simulink library "exampleMicrogridLibrary"  (R2017b)
settings: Solver=VariableStepAuto  StartTime=0.0  StopTime=10.0  RelTol=1e-3
undefined symbols (not defined in the file): BR, D1, Delta, DiscIntNeverNeededParam, Fnom, gcbh, Ion, kv, Lithium, Ls, Rs, sps_rtmsupport, StationData, Ts, Ts_Control, Vrms
libraries: powerlib x75, simulink x29, powerlib_meascontrol x26, sps_avr x5, spsDieselMotorModel x3, electricdrivelib x2, re_lib x1
(part 5 of 5)

== system exampleMicrogridLibrary/Solar Array (EMT Model)/Inverter Control/Current Regulator ==
  note: Current Regulator
      | ================
  note: Sign Convention: Current going out of the converter = positive current
  note: Iq positive --> The converter absorbs reactive power ("Inductive mode") = Reactive Power Q negative
  note: Id positive --> The converter generates active power ("Inverter mode") = Active Power P positive
  VdVq_meas : Inport  PortDimensions=2
  IdIq_meas : Inport  Port=2  PortDimensions=2
  IdIq_ref : Inport  Port=3  PortDimensions=2
  Add1 : Sum  Inputs=++-
  Add2 : Sum
  Add3 : Sum  Inputs=+++
  Demux : Demux  Outputs=2
  Demux1 : Demux  Outputs=2
  Lff : Gain  Gain=Ltot_pu  SaturateOnIntegerOverflow=on  OutDataTypeStr=Inherit: Same as input  ParamDataTypeStr=Inherit: Same as input
  "Lff  " : Gain  Gain=Ltot_pu  SaturateOnIntegerOverflow=on  OutDataTypeStr=Inherit: Same as input  ParamDataTypeStr=Inherit: Same as input
  Mux : Mux  Inputs=2
  PI : simulink/Continuous/PID Controller  Controller=PI  TimeDomain=Discrete-time  SampleTime=Ts_Control  IntegratorMethod=Forward Euler  FilterMethod=Forward Euler  Form=Parallel  UseFilter=on  ControllerParametersSource=internal  P=Kp_Ireg  I=Ki_Ireg  D=0  N=100  InitialConditionSource=internal  InitialConditionForIntegrator=0  InitialConditionForFilter=0  ExternalReset=none  LimitOutput=on  UpperSaturationLimit=1.5  LowerSaturationLimit=-1.5  LinearizeAsGain=off  AntiWindupMode=none  Kb=1  TrackingMode=off  Kt=1  PParamMin=[]  PParamMax=[]  IParamMin=[]  IParamMax=[]  DParamMin=[]  DParamMax=[]  NParamMin=[]  NParamMax=[]  KbParamMin=[]  KbParamMax=[]  KtParamMin=[]  KtParamMax=[]  POutMin=[]  POutMax=[]  IOutMin=[]  IOutMax=[]  DOutMin=[]  DOutMax=[]  NOutMin=[]  NOutMax=[]  KbOutMin=[]  KbOutMax=[]  KtOutMin=[]  KtOutMax=[]  IntegratorOutMin=[]  IntegratorOutMax=[]  FilterOutMin=[]  FilterOutMax=[]  SumOutMin=[]  SumOutMax=[]  SumI1OutMin=[]  SumI1OutMax=[]  SumI2OutMin=[]  SumI2OutMax=[]  SumI3OutMin=[]  SumI3OutMax=[]  SumDOutMin=[]  SumDOutMax=[]  SaturationOutMin=[]  SaturationOutMax=[]  IntegratorContinuousStateAttributes=''  IntegratorStateMustResolveToSignalObject=off  IntegratorRTWStateStorageClass=Auto  FilterContinuousStateAttributes=''  FilterStateMustResolveToSignalObject=off  FilterRTWStateStorageClass=Auto  DifferentiatorICPrevScaledInput=0  DifferentiatorOutMin=[]  DifferentiatorOutMax=[]  InitialConditionSetting=State (most efficient)  FilterDiffOutCoefMin=[]  FilterDiffOutCoefMax=[]  SumDenOutMin=[]  SumDenOutMax=[]  SumNumOutMin=[]  SumNumOutMax=[]  ReciprocalOutMin=[]  ReciprocalOutMax=[]  DivideOutMin=[]  DivideOutMax=[]  TunerSelectOption=Transfer Function Based (PID Tuner App)
  Rff : Gain  Gain=Rtot_pu  SaturateOnIntegerOverflow=on  OutDataTypeStr=Inherit: Same as input  ParamDataTypeStr=Inherit: Same as input
  "Rff " : Gain  Gain=Rtot_pu  SaturateOnIntegerOverflow=on  OutDataTypeStr=Inherit: Same as input  ParamDataTypeStr=Inherit: Same as input
  Saturation : Saturate  UpperLimit=1.5  LowerLimit=-1.5
  Sum : Sum  Inputs=|-+
  VdVq_conv : Outport
  wires:
  Mux/1 -> Add2/2
  PI/1 -> Add2/1  "PI"
  Sum/1 -> PI/1
  IdIq_ref/1 -> Sum/2, Demux1/1
  IdIq_meas/1 -> Sum/1
  Add2/1 -> Saturation/1
  Saturation/1 -> VdVq_conv/1
  VdVq_meas/1 -> Demux/1
  Demux/1 -> Add1/1
  "Rff "/1 -> Add1/2
  Demux1/1 -> "Rff "/1, Lff/1
  "Lff  "/1 -> Add1/3
  Demux1/2 -> "Lff  "/1, Rff/1
  Rff/1 -> Add3/2
  Lff/1 -> Add3/3
  Add1/1 -> Mux/1  "Feedforward"
  Demux/2 -> Add3/1
  Add3/1 -> Mux/2

== system exampleMicrogridLibrary/Solar Array (EMT Model)/Inverter Control/MPPT Parameters ==
  note: Parameters for Perturb and Observe Algorithm:
  note: Lower limit for Vdc_ref (Dmax)
  note: Initial value for Vdc_ref output (Dinit)
  note: Increment value used to increase/decrease Vdc_ref (DeltaD)
  note: Upper limit for Vdc_ref (Dmax)
  Iph_ : Constant  Value=Vnom_dc
  Iph_1 : Constant  Value=Limits_MPPT(1)
  Iph_2 : Constant  Value=Limits_MPPT(2)
  Iph_3 : Constant  Value=Increment_MPPT
  Mux : Mux
  Param : Outport
  wires:
  Mux/1 -> Param/1
  Iph_3/1 -> Mux/4
  Iph_2/1 -> Mux/3
  Iph_1/1 -> Mux/2
  Iph_/1 -> Mux/1

== system exampleMicrogridLibrary/Solar Array (EMT Model)/Inverter Control/PLL & Measurements ==
  note: PLL & Measurements
      | ===================
  Vabc_prim : Inport
  Iabc_prim : Inport  Port=2
  PLL (3ph) : powerlib_meascontrol/PLL/PLL (3ph)  Fmin=45  Par_Init="[-0.57  Fnom]"  ParK=[180, 3200, 1]  TcD=Ts  MaxRateChangeFreq=12  FilterCutOffFreq=25  Ts=Ts  AGC=on
  Selector1 : Selector  InputPortWidth=3  IndexOptions=Index vector (dialog)  Indices=[1 2]  OutputSizes=1
  Selector2 : Selector  InputPortWidth=3  IndexOptions=Index vector (dialog)  Indices=[1 2]  OutputSizes=1
  Terminator : Terminator
  V->pu : Gain  Gain=1/(Vnom_prim*sqrt(2)/sqrt(3))  SaturateOnIntegerOverflow=on  OutDataTypeStr=Inherit: Same as input  ParamDataTypeStr=Inherit: Same as input
  V->pu1 : Gain  Gain=Vnom_prim*sqrt(3)/Pnom/sqrt(2)  SaturateOnIntegerOverflow=on  OutDataTypeStr=Inherit: Same as input  ParamDataTypeStr=Inherit: Same as input
  abc to dq0 : powerlib_meascontrol/Transformations/abc to dq0  Alignment=90 degrees behind phase A axis
  abc to dq1 : powerlib_meascontrol/Transformations/abc to dq0  Alignment=90 degrees behind phase A axis
  wt : Outport
  VdVq_prim : Outport  Port=2
  IdIq_prim : Outport  Port=3
  wires:
  V->pu1/1 -> abc to dq1/1
  V->pu/1 -> PLL (3ph)/1, abc to dq0/1
  abc to dq1/1 -> Selector1/1
  Vabc_prim/1 -> V->pu/1
  Iabc_prim/1 -> V->pu1/1
  abc to dq0/1 -> Selector2/1
  Selector2/1 -> VdVq_prim/1
  Selector1/1 -> IdIq_prim/1
  PLL (3ph)/2 -> wt/1, abc to dq1/2, abc to dq0/2
  PLL (3ph)/1 -> Terminator/1

== system exampleMicrogridLibrary/Solar Array (EMT Model)/Inverter Control/Uabc_ref Generation max (m) = 1 ==
  note: (Correction for transformer
      |  D1 connection)
  note: (Correction for delai of Ts_Control)
  note: Uref Generation
      | ==============
  wt : Inport
  VdVq_conv : Inport  Port=2
  Add1 : Sum  Inputs=++++
  Add2 : Sum
  Complex to Magnitude-Angle : ComplexToMagnitudeAngle
  Constant : Constant  Value=-pi/6
  Constant1 : Constant  Value=Vnom_dc
  Constant2 : Constant  Value="[ 0  -2*pi/3  2*pi/3  ]"
  Constant3 : Constant  Value=Vnom_sec*sqrt(2)/sqrt(3)
  Constant4 : Constant  Value=Ts_Control*Fnom*(2*pi)
  Demux1 : Demux  Outputs=2
  Gain1 : Gain  Gain=1/2
  Product : Product  Inputs=*/  RndMeth=Zero
  Product1 : Product  Inputs=*/  RndMeth=Zero
  Product2 : Product  Inputs=**  RndMeth=Zero
  Real-Imag to Complex : RealImagToComplex
  Trigonometric Function : Trigonometry
  Uabc_ref : Outport
  wires:
  Constant1/1 -> Gain1/1
  VdVq_conv/1 -> Product1/1
  Product1/1 -> Demux1/1
  Gain1/1 -> Product/1
  Real-Imag to Complex/1 -> Complex to Magnitude-Angle/1
  Demux1/1 -> Real-Imag to Complex/1
  Demux1/2 -> Real-Imag to Complex/2
  Constant2/1 -> Add1/2
  Constant/1 -> Add1/3
  Constant3/1 -> Product/2
  Product/1 -> Product1/2
  Complex to Magnitude-Angle/2 -> Add2/1
  Add1/1 -> Add2/2
  Add2/1 -> Trigonometric Function/1
  Complex to Magnitude-Angle/1 -> Product2/1
  Trigonometric Function/1 -> Product2/2
  Product2/1 -> Uabc_ref/1
  wt/1 -> Add1/1
  Constant4/1 -> Add1/4

== system exampleMicrogridLibrary/Solar Array (EMT Model)/Inverter Control/VDC Regulator ==
  Vdc_meas : Inport  PortDimensions=1
  Vdc_ref : Inport  Port=2  PortDimensions=1
  PI : simulink/Continuous/PID Controller  Controller=PI  TimeDomain=Discrete-time  SampleTime=Ts_Control  IntegratorMethod=Trapezoidal  FilterMethod=Forward Euler  Form=Parallel  UseFilter=on  ControllerParametersSource=internal  P=Kp_VDCreg  I=Ki_VDCreg  D=0  N=100  InitialConditionSource=internal  InitialConditionForIntegrator=1  InitialConditionForFilter=0  ExternalReset=none  LimitOutput=on  UpperSaturationLimit=1.5  LowerSaturationLimit=-1.5  LinearizeAsGain=off  AntiWindupMode=none  Kb=1  TrackingMode=off  Kt=1  PParamMin=[]  PParamMax=[]  IParamMin=[]  IParamMax=[]  DParamMin=[]  DParamMax=[]  NParamMin=[]  NParamMax=[]  KbParamMin=[]  KbParamMax=[]  KtParamMin=[]  KtParamMax=[]  POutMin=[]  POutMax=[]  IOutMin=[]  IOutMax=[]  DOutMin=[]  DOutMax=[]  NOutMin=[]  NOutMax=[]  KbOutMin=[]  KbOutMax=[]  KtOutMin=[]  KtOutMax=[]  IntegratorOutMin=[]  IntegratorOutMax=[]  FilterOutMin=[]  FilterOutMax=[]  SumOutMin=[]  SumOutMax=[]  SumI1OutMin=[]  SumI1OutMax=[]  SumI2OutMin=[]  SumI2OutMax=[]  SumI3OutMin=[]  SumI3OutMax=[]  SumDOutMin=[]  SumDOutMax=[]  SaturationOutMin=[]  SaturationOutMax=[]  IntegratorContinuousStateAttributes=''  IntegratorStateMustResolveToSignalObject=off  IntegratorRTWStateStorageClass=Auto  FilterContinuousStateAttributes=''  FilterStateMustResolveToSignalObject=off  FilterRTWStateStorageClass=Auto  DifferentiatorICPrevScaledInput=0  DifferentiatorOutMin=[]  DifferentiatorOutMax=[]  InitialConditionSetting=State (most efficient)  FilterDiffOutCoefMin=[]  FilterDiffOutCoefMax=[]  SumDenOutMin=[]  SumDenOutMax=[]  SumNumOutMin=[]  SumNumOutMax=[]  ReciprocalOutMin=[]  ReciprocalOutMax=[]  DivideOutMin=[]  DivideOutMax=[]  TunerSelectOption=Transfer Function Based (PID Tuner App)
  Rtot_pu3 : Gain  Gain=1/Vnom_dc  SaturateOnIntegerOverflow=on  OutDataTypeStr=Inherit: Same as input  ParamDataTypeStr=Inherit: Same as input
  Sum : Sum  Inputs=|+-
  Id_ref : Outport  InitialOutput=0
  wires:
  PI/1 -> Id_ref/1
  Rtot_pu3/1 -> PI/1
  Vdc_ref/1 -> Sum/2
  Vdc_meas/1 -> Sum/1
  Sum/1 -> Rtot_pu3/1

== system exampleMicrogridLibrary/Diesel Generator (Full Genset Controls)/Continuous/Automatic Generator Controls/PQ Control ==
  PQ_wv_ref : Inport
  GenM : Inport  Port=2
  Bus Selector1 : BusSelector  OutputSignals=Active Power (W)
  Bus Selector2 : BusSelector  OutputSignals=Reactive Power (W)
  Exciter Controller : simulink/Continuous/PID Controller  Controller=PI  TimeDomain=Continuous-time  SampleTime=-1  IntegratorMethod=Forward Euler  FilterMethod=Forward Euler  Form=Parallel  UseFilter=on  ControllerParametersSource=internal  P=1  I=0.1  D=0  N=100  InitialConditionSource=internal  InitialConditionForIntegrator=1  InitialConditionForFilter=0  ExternalReset=none  ZeroCross=off  LimitOutput=on  UpperSaturationLimit=1.005  LowerSaturationLimit=0.995  LinearizeAsGain=on  AntiWindupMode=clamping  Kb=1  TrackingMode=off  Kt=1  PParamMin=[]  PParamMax=[]  IParamMin=[]  IParamMax=[]  DParamMin=[]  DParamMax=[]  NParamMin=[]  NParamMax=[]  KbParamMin=[]  KbParamMax=[]  KtParamMin=[]  KtParamMax=[]  POutMin=[]  POutMax=[]  IOutMin=[]  IOutMax=[]  DOutMin=[]  DOutMax=[]  NOutMin=[]  NOutMax=[]  KbOutMin=[]  KbOutMax=[]  KtOutMin=[]  KtOutMax=[]  IntegratorOutMin=[]  IntegratorOutMax=[]  FilterOutMin=[]  FilterOutMax=[]  SumOutMin=[]  SumOutMax=[]  SumI1OutMin=[]  SumI1OutMax=[]  SumI2OutMin=[]  SumI2OutMax=[]  SumI3OutMin=[]  SumI3OutMax=[]  SumDOutMin=[]  SumDOutMax=[]  SaturationOutMin=[]  SaturationOutMax=[]  IntegratorContinuousStateAttributes=''  IntegratorStateMustResolveToSignalObject=off  IntegratorRTWStateStorageClass=Auto  FilterContinuousStateAttributes=''  FilterStateMustResolveToSignalObject=off  FilterRTWStateStorageClass=Auto  DifferentiatorICPrevScaledInput=0  DifferentiatorOutMin=[]  DifferentiatorOutMax=[]  InitialConditionSetting=State (most efficient)  FilterDiffOutCoefMin=[]  FilterDiffOutCoefMax=[]  SumDenOutMin=[]  SumDenOutMax=[]  SumNumOutMin=[]  SumNumOutMax=[]  ReciprocalOutMin=[]  ReciprocalOutMax=[]  DivideOutMin=[]  DivideOutMax=[]  TunerSelectOption=Transfer Function Based (PID Tuner App)
  GenM1 : InportShadow  Port=2
  Governor Controller : simulink/Continuous/PID Controller  Controller=I  TimeDomain=Continuous-time  SampleTime=-1  IntegratorMethod=Forward Euler  FilterMethod=Forward Euler  Form=Parallel  UseFilter=on  ControllerParametersSource=internal  P=1e-6  I=0.3  D=0  N=100  InitialConditionSource=internal  InitialConditionForIntegrator=1  InitialConditionForFilter=0  ExternalReset=none  ZeroCross=off  LimitOutput=on  UpperSaturationLimit=1.005  LowerSaturationLimit=0.995  LinearizeAsGain=on  AntiWindupMode=clamping  Kb=1  TrackingMode=off  Kt=1  PParamMin=[]  PParamMax=[]  IParamMin=[]  IParamMax=[]  DParamMin=[]  DParamMax=[]  NParamMin=[]  NParamMax=[]  KbParamMin=[]  KbParamMax=[]  KtParamMin=[]  KtParamMax=[]  POutMin=[]  POutMax=[]  IOutMin=[]  IOutMax=[]  DOutMin=[]  DOutMax=[]  NOutMin=[]  NOutMax=[]  KbOutMin=[]  KbOutMax=[]  KtOutMin=[]  KtOutMax=[]  IntegratorOutMin=[]  IntegratorOutMax=[]  FilterOutMin=[]  FilterOutMax=[]  SumOutMin=[]  SumOutMax=[]  SumI1OutMin=[]  SumI1OutMax=[]  SumI2OutMin=[]  SumI2OutMax=[]  SumI3OutMin=[]  SumI3OutMax=[]  SumDOutMin=[]  SumDOutMax=[]  SaturationOutMin=[]  SaturationOutMax=[]  IntegratorContinuousStateAttributes=''  IntegratorStateMustResolveToSignalObject=off  IntegratorRTWStateStorageClass=Auto  FilterContinuousStateAttributes=''  FilterStateMustResolveToSignalObject=off  FilterRTWStateStorageClass=Auto  DifferentiatorICPrevScaledInput=0  DifferentiatorOutMin=[]  DifferentiatorOutMax=[]  InitialConditionSetting=State (most efficient)  FilterDiffOutCoefMin=[]  FilterDiffOutCoefMax=[]  SumDenOutMin=[]  SumDenOutMax=[]  SumNumOutMin=[]  SumNumOutMax=[]  ReciprocalOutMin=[]  ReciprocalOutMax=[]  DivideOutMin=[]  DivideOutMax=[]  TunerSelectOption=Transfer Function Based (PID Tuner App)
  Mux : Mux  Inputs=2
  PQ_wv_ref1 : InportShadow
  Selector : Selector  InputPortWidth=4  IndexOptions=Index vector (dialog)  Indices=[1]  OutputSizes=1
  Selector1 : Selector  InputPortWidth=4  IndexOptions=Index vector (dialog)  Indices=[2]  OutputSizes=1
  Sum1 : Sum  Inputs=|+-
  Sum2 : Sum  Inputs=|+-
  to PU : Gain  Gain=1/Pn
  to PU1 : Gain  Gain=1/Pn
  "wref, Vref" : Outport
  wires:
  Mux/1 -> "wref, Vref"/1
  Governor Controller/1 -> Mux/1
  to PU1/1 -> Exciter Controller/1
  Sum2/1 -> to PU/1
  to PU/1 -> Governor Controller/1
  Sum1/1 -> to PU1/1
  Selector1/1 -> Sum1/1  "Qref"
  Selector/1 -> Sum2/1  "Pref"
  Bus Selector1/1 -> Sum2/2  "<Active Power (W)>"
  GenM1/1 -> Bus Selector2/1
  GenM/1 -> Bus Selector1/1
  Bus Selector2/1 -> Sum1/2  "<Reactive Power (W)>"
  Exciter Controller/1 -> Mux/2
  PQ_wv_ref/1 -> Selector/1
  PQ_wv_ref1/1 -> Selector1/1

== system exampleMicrogridLibrary/Diesel Generator (Full Genset Controls)/Continuous/Automatic Generator Controls/PV Control ==
  PQ_wv_ref : Inport
  GenM : Inport  Port=2
  Bus Selector1 : BusSelector  OutputSignals=Active Power (W)
  Governor Controller : simulink/Continuous/PID Controller  Controller=I  TimeDomain=Continuous-time  SampleTime=-1  IntegratorMethod=Forward Euler  FilterMethod=Forward Euler  Form=Parallel  UseFilter=on  ControllerParametersSource=internal  P=1e-6  I=0.3  D=0  N=100  InitialConditionSource=internal  InitialConditionForIntegrator=1  InitialConditionForFilter=0  ExternalReset=none  ZeroCross=off  LimitOutput=on  UpperSaturationLimit=1.005  LowerSaturationLimit=0.995  LinearizeAsGain=on  AntiWindupMode=clamping  Kb=1  TrackingMode=off  Kt=1  PParamMin=[]  PParamMax=[]  IParamMin=[]  IParamMax=[]  DParamMin=[]  DParamMax=[]  NParamMin=[]  NParamMax=[]  KbParamMin=[]  KbParamMax=[]  KtParamMin=[]  KtParamMax=[]  POutMin=[]  POutMax=[]  IOutMin=[]  IOutMax=[]  DOutMin=[]  DOutMax=[]  NOutMin=[]  NOutMax=[]  KbOutMin=[]  KbOutMax=[]  KtOutMin=[]  KtOutMax=[]  IntegratorOutMin=[]  IntegratorOutMax=[]  FilterOutMin=[]  FilterOutMax=[]  SumOutMin=[]  SumOutMax=[]  SumI1OutMin=[]  SumI1OutMax=[]  SumI2OutMin=[]  SumI2OutMax=[]  SumI3OutMin=[]  SumI3OutMax=[]  SumDOutMin=[]  SumDOutMax=[]  SaturationOutMin=[]  SaturationOutMax=[]  IntegratorContinuousStateAttributes=''  IntegratorStateMustResolveToSignalObject=off  IntegratorRTWStateStorageClass=Auto  FilterContinuousStateAttributes=''  FilterStateMustResolveToSignalObject=off  FilterRTWStateStorageClass=Auto  DifferentiatorICPrevScaledInput=0  DifferentiatorOutMin=[]  DifferentiatorOutMax=[]  InitialConditionSetting=State (most efficient)  FilterDiffOutCoefMin=[]  FilterDiffOutCoefMax=[]  SumDenOutMin=[]  SumDenOutMax=[]  SumNumOutMin=[]  SumNumOutMax=[]  ReciprocalOutMin=[]  ReciprocalOutMax=[]  DivideOutMin=[]  DivideOutMax=[]  TunerSelectOption=Transfer Function Based (PID Tuner App)
  Mux : Mux  Inputs=2
  PQ_wv_ref1 : InportShadow
  Selector : Selector  InputPortWidth=4  IndexOptions=Index vector (dialog)  Indices=[1]  OutputSizes=1
  Selector1 : Selector  InputPortWidth=4  IndexOptions=Index vector (dialog)  Indices=[4]  OutputSizes=1
  Sum2 : Sum  Inputs=|+-
  to PU : Gain  Gain=1/Pn
  "wref, Vref" : Outport
  wires:
  PQ_wv_ref1/1 -> Selector1/1
  PQ_wv_ref/1 -> Selector/1
  Selector1/1 -> Mux/2  "Vref"
  GenM/1 -> Bus Selector1/1
  Bus Selector1/1 -> Sum2/2  "<Active Power (W)>"
  Selector/1 -> Sum2/1  "Pref"
  to PU/1 -> Governor Controller/1
  Sum2/1 -> to PU/1
  Governor Controller/1 -> Mux/1
  Mux/1 -> "wref, Vref"/1

== system exampleMicrogridLibrary/Diesel Generator (Full Genset Controls)/Discrete/Automatic Generator Controls/PQ Control ==
  PQ_wv_ref : Inport
  GenM : Inport  Port=2
  Bus Selector1 : BusSelector  OutputSignals=Active Power (W)
  Bus Selector2 : BusSelector  OutputSignals=Reactive Power (W)
  Exciter Controller : simulink/Continuous/PID Controller  Controller=PI  TimeDomain=Discrete-time  SampleTime=Ts  IntegratorMethod=Forward Euler  FilterMethod=Forward Euler  Form=Parallel  UseFilter=on  ControllerParametersSource=internal  P=1  I=0.1  D=0  N=100  InitialConditionSource=internal  InitialConditionForIntegrator=1  InitialConditionForFilter=0  ExternalReset=none  ZeroCross=off  LimitOutput=on  UpperSaturationLimit=1.005  LowerSaturationLimit=0.995  LinearizeAsGain=on  AntiWindupMode=clamping  Kb=1  TrackingMode=off  Kt=1  PParamMin=[]  PParamMax=[]  IParamMin=[]  IParamMax=[]  DParamMin=[]  DParamMax=[]  NParamMin=[]  NParamMax=[]  KbParamMin=[]  KbParamMax=[]  KtParamMin=[]  KtParamMax=[]  POutMin=[]  POutMax=[]  IOutMin=[]  IOutMax=[]  DOutMin=[]  DOutMax=[]  NOutMin=[]  NOutMax=[]  KbOutMin=[]  KbOutMax=[]  KtOutMin=[]  KtOutMax=[]  IntegratorOutMin=[]  IntegratorOutMax=[]  FilterOutMin=[]  FilterOutMax=[]  SumOutMin=[]  SumOutMax=[]  SumI1OutMin=[]  SumI1OutMax=[]  SumI2OutMin=[]  SumI2OutMax=[]  SumI3OutMin=[]  SumI3OutMax=[]  SumDOutMin=[]  SumDOutMax=[]  SaturationOutMin=[]  SaturationOutMax=[]  IntegratorContinuousStateAttributes=''  IntegratorStateMustResolveToSignalObject=off  IntegratorRTWStateStorageClass=Auto  FilterContinuousStateAttributes=''  FilterStateMustResolveToSignalObject=off  FilterRTWStateStorageClass=Auto  DifferentiatorICPrevScaledInput=0  DifferentiatorOutMin=[]  DifferentiatorOutMax=[]  InitialConditionSetting=State (most efficient)  FilterDiffOutCoefMin=[]  FilterDiffOutCoefMax=[]  SumDenOutMin=[]  SumDenOutMax=[]  SumNumOutMin=[]  SumNumOutMax=[]  ReciprocalOutMin=[]  ReciprocalOutMax=[]  DivideOutMin=[]  DivideOutMax=[]  TunerSelectOption=Transfer Function Based (PID Tuner App)
  GenM1 : InportShadow  Port=2
  Governor Controller : simulink/Continuous/PID Controller  Controller=I  TimeDomain=Discrete-time  SampleTime=Ts  IntegratorMethod=Forward Euler  FilterMethod=Forward Euler  Form=Parallel  UseFilter=on  ControllerParametersSource=internal  P=1e-6  I=0.3  D=0  N=100  InitialConditionSource=internal  InitialConditionForIntegrator=1  InitialConditionForFilter=0  ExternalReset=none  ZeroCross=off  LimitOutput=on  UpperSaturationLimit=1.005  LowerSaturationLimit=0.995  LinearizeAsGain=on  AntiWindupMode=clamping  Kb=1  TrackingMode=off  Kt=1  PParamMin=[]  PParamMax=[]  IParamMin=[]  IParamMax=[]  DParamMin=[]  DParamMax=[]  NParamMin=[]  NParamMax=[]  KbParamMin=[]  KbParamMax=[]  KtParamMin=[]  KtParamMax=[]  POutMin=[]  POutMax=[]  IOutMin=[]  IOutMax=[]  DOutMin=[]  DOutMax=[]  NOutMin=[]  NOutMax=[]  KbOutMin=[]  KbOutMax=[]  KtOutMin=[]  KtOutMax=[]  IntegratorOutMin=[]  IntegratorOutMax=[]  FilterOutMin=[]  FilterOutMax=[]  SumOutMin=[]  SumOutMax=[]  SumI1OutMin=[]  SumI1OutMax=[]  SumI2OutMin=[]  SumI2OutMax=[]  SumI3OutMin=[]  SumI3OutMax=[]  SumDOutMin=[]  SumDOutMax=[]  SaturationOutMin=[]  SaturationOutMax=[]  IntegratorContinuousStateAttributes=''  IntegratorStateMustResolveToSignalObject=off  IntegratorRTWStateStorageClass=Auto  FilterContinuousStateAttributes=''  FilterStateMustResolveToSignalObject=off  FilterRTWStateStorageClass=Auto  DifferentiatorICPrevScaledInput=0  DifferentiatorOutMin=[]  DifferentiatorOutMax=[]  InitialConditionSetting=State (most efficient)  FilterDiffOutCoefMin=[]  FilterDiffOutCoefMax=[]  SumDenOutMin=[]  SumDenOutMax=[]  SumNumOutMin=[]  SumNumOutMax=[]  ReciprocalOutMin=[]  ReciprocalOutMax=[]  DivideOutMin=[]  DivideOutMax=[]  TunerSelectOption=Transfer Function Based (PID Tuner App)
  Mux : Mux  Inputs=2
  PQ_wv_ref1 : InportShadow
  Selector : Selector  InputPortWidth=4  IndexOptions=Index vector (dialog)  Indices=[1]  OutputSizes=1
  Selector1 : Selector  InputPortWidth=4  IndexOptions=Index vector (dialog)  Indices=[2]  OutputSizes=1
  Sum1 : Sum  Inputs=|+-
  Sum2 : Sum  Inputs=|+-
  to PU : Gain  Gain=1/Pn
  to PU1 : Gain  Gain=1/Pn
  "wref, Vref" : Outport
  wires:
  Mux/1 -> "wref, Vref"/1
  Governor Controller/1 -> Mux/1
  to PU1/1 -> Exciter Controller/1
  Sum2/1 -> to PU/1
  to PU/1 -> Governor Controller/1
  Sum1/1 -> to PU1/1
  Selector1/1 -> Sum1/1  "Qref"
  Selector/1 -> Sum2/1  "Pref"
  Bus Selector1/1 -> Sum2/2  "<Active Power (W)>"
  GenM1/1 -> Bus Selector2/1
  GenM/1 -> Bus Selector1/1
  Bus Selector2/1 -> Sum1/2  "<Reactive Power (W)>"
  Exciter Controller/1 -> Mux/2
  PQ_wv_ref/1 -> Selector/1
  PQ_wv_ref1/1 -> Selector1/1

== system exampleMicrogridLibrary/Diesel Generator (Full Genset Controls)/Discrete/Automatic Generator Controls/PV Control ==
  PQ_wv_ref : Inport
  GenM : Inport  Port=2
  Bus Selector1 : BusSelector  OutputSignals=Active Power (W)
  Governor Controller : simulink/Continuous/PID Controller  Controller=I  TimeDomain=Discrete-time  SampleTime=Ts  IntegratorMethod=Forward Euler  FilterMethod=Forward Euler  Form=Parallel  UseFilter=on  ControllerParametersSource=internal  P=1e-6  I=0.3  D=0  N=100  InitialConditionSource=internal  InitialConditionForIntegrator=1  InitialConditionForFilter=0  ExternalReset=none  ZeroCross=off  LimitOutput=on  UpperSaturationLimit=1.005  LowerSaturationLimit=0.995  LinearizeAsGain=on  AntiWindupMode=clamping  Kb=1  TrackingMode=off  Kt=1  PParamMin=[]  PParamMax=[]  IParamMin=[]  IParamMax=[]  DParamMin=[]  DParamMax=[]  NParamMin=[]  NParamMax=[]  KbParamMin=[]  KbParamMax=[]  KtParamMin=[]  KtParamMax=[]  POutMin=[]  POutMax=[]  IOutMin=[]  IOutMax=[]  DOutMin=[]  DOutMax=[]  NOutMin=[]  NOutMax=[]  KbOutMin=[]  KbOutMax=[]  KtOutMin=[]  KtOutMax=[]  IntegratorOutMin=[]  IntegratorOutMax=[]  FilterOutMin=[]  FilterOutMax=[]  SumOutMin=[]  SumOutMax=[]  SumI1OutMin=[]  SumI1OutMax=[]  SumI2OutMin=[]  SumI2OutMax=[]  SumI3OutMin=[]  SumI3OutMax=[]  SumDOutMin=[]  SumDOutMax=[]  SaturationOutMin=[]  SaturationOutMax=[]  IntegratorContinuousStateAttributes=''  IntegratorStateMustResolveToSignalObject=off  IntegratorRTWStateStorageClass=Auto  FilterContinuousStateAttributes=''  FilterStateMustResolveToSignalObject=off  FilterRTWStateStorageClass=Auto  DifferentiatorICPrevScaledInput=0  DifferentiatorOutMin=[]  DifferentiatorOutMax=[]  InitialConditionSetting=State (most efficient)  FilterDiffOutCoefMin=[]  FilterDiffOutCoefMax=[]  SumDenOutMin=[]  SumDenOutMax=[]  SumNumOutMin=[]  SumNumOutMax=[]  ReciprocalOutMin=[]  ReciprocalOutMax=[]  DivideOutMin=[]  DivideOutMax=[]  TunerSelectOption=Transfer Function Based (PID Tuner App)
  Mux : Mux  Inputs=2
  PQ_wv_ref1 : InportShadow
  Selector : Selector  InputPortWidth=4  IndexOptions=Index vector (dialog)  Indices=[1]  OutputSizes=1
  Selector1 : Selector  InputPortWidth=4  IndexOptions=Index vector (dialog)  Indices=[4]  OutputSizes=1
  Sum2 : Sum  Inputs=|+-
  to PU : Gain  Gain=1/Pn
  "wref, Vref" : Outport
  wires:
  PQ_wv_ref1/1 -> Selector1/1
  PQ_wv_ref/1 -> Selector/1
  Selector1/1 -> Mux/2  "Vref"
  GenM/1 -> Bus Selector1/1
  Bus Selector1/1 -> Sum2/2  "<Active Power (W)>"
  Selector/1 -> Sum2/1  "Pref"
  to PU/1 -> Governor Controller/1
  Sum2/1 -> to PU/1
  Governor Controller/1 -> Mux/1
  Mux/1 -> "wref, Vref"/1

== system exampleMicrogridLibrary/Diesel Generator (Full Genset Controls)/Discrete/Diesel Engine Governor/CONTROL SYSTEM ==
  In1 : Inport
  Discrete-Time Integrator1 : DiscreteIntegrator  SampleTime=Ts  ICPrevOutput=DiscIntNeverNeededParam  ICPrevScaledInput=DiscIntNeverNeededParam
  Discrete-Time Integrator2 : DiscreteIntegrator  SampleTime=Ts  ICPrevOutput=DiscIntNeverNeededParam  ICPrevScaledInput=DiscIntNeverNeededParam
  Gain2 : Gain  Gain=1/Tr(2)
  Gain3 : Gain  Gain=1/(Tr(1)*Tr(2))
  Gain4 : Gain  Gain=Tr(3)
  Gain7 : Gain  Gain=1/(Tr(1)*Tr(2))
  Sum2 : Sum  Inputs=|+-
  Sum3 : Sum  Inputs=|++
  Sum4 : Sum  Inputs=++|
  Out1 : Outport
  wires:
  Gain4/1 -> Sum4/1
  Sum4/1 -> Out1/1
  Discrete-Time Integrator1/1 -> Gain3/1, Sum4/2
  Sum3/1 -> Sum2/2  "Vs0/A2"
  Gain7/1 -> Sum2/1
  Gain3/1 -> Sum3/1
  Gain2/1 -> Sum3/2
  Sum2/1 -> Discrete-Time Integrator2/1
  Discrete-Time Integrator2/1 -> Gain4/1, Gain2/1, Discrete-Time Integrator1/1
  In1/1 -> Gain7/1

== system exampleMicrogridLibrary/Diesel Generator (Full Genset Controls)/Discrete/Diesel Engine Governor/TF1 ==
  In1 : Inport
  Discrete-Time Integrator : DiscreteIntegrator  SampleTime=Ts  ICPrevOutput=DiscIntNeverNeededParam  ICPrevScaledInput=DiscIntNeverNeededParam
  Gain : Gain  Gain=1/Ta(2)
  Gain1 : Gain  Gain=Ta(1)
  Sum1 : Sum  Inputs=|+-
  Sum2 : Sum  Inputs=++|
  Out1 : Outport
  wires:
  Sum2/1 -> Out1/1
  Sum1/1 -> Gain/1
  Gain1/1 -> Sum2/1
  Discrete-Time Integrator/1 -> Sum1/2, Sum2/2
  In1/1 -> Sum1/1
  Gain/1 -> Gain1/1, Discrete-Time Integrator/1

== system exampleMicrogridLibrary/Diesel Generator (Full Genset Controls)/Discrete/Diesel Engine Governor/TF2 ==
  In1 : Inport
  1/T6 : Gain  Gain=1/Ta(3)
  Discrete-Time Integrator : DiscreteIntegrator  SampleTime=Ts  ICPrevOutput=DiscIntNeverNeededParam  ICPrevScaledInput=DiscIntNeverNeededParam
  Sum1 : Sum  Inputs=|+-
  Out1 : Outport
  wires:
  Sum1/1 -> 1/T6/1
  Discrete-Time Integrator/1 -> Sum1/2, Out1/1
  In1/1 -> Sum1/1
  1/T6/1 -> Discrete-Time Integrator/1

== system exampleMicrogridLibrary/Diesel Generator (Simple Controls)/Discrete/Diesel Engine Governor/CONTROL SYSTEM ==
  In1 : Inport
  Discrete-Time Integrator1 : DiscreteIntegrator  SampleTime=Ts  ICPrevOutput=DiscIntNeverNeededParam  ICPrevScaledInput=DiscIntNeverNeededParam
  Discrete-Time Integrator2 : DiscreteIntegrator  SampleTime=Ts  ICPrevOutput=DiscIntNeverNeededParam  ICPrevScaledInput=DiscIntNeverNeededParam
  Gain2 : Gain  Gain=1/Tr(2)
  Gain3 : Gain  Gain=1/(Tr(1)*Tr(2))
  Gain4 : Gain  Gain=Tr(3)
  Gain7 : Gain  Gain=1/(Tr(1)*Tr(2))
  Sum2 : Sum  Inputs=|+-
  Sum3 : Sum  Inputs=|++
  Sum4 : Sum  Inputs=++|
  Out1 : Outport
  wires:
  In1/1 -> Gain7/1
  Discrete-Time Integrator2/1 -> Discrete-Time Integrator1/1, Gain2/1, Gain4/1
  Sum2/1 -> Discrete-Time Integrator2/1
  Gain2/1 -> Sum3/2
  Gain3/1 -> Sum3/1
  Gain7/1 -> Sum2/1
  Sum3/1 -> Sum2/2  "Vs0/A2"
  Discrete-Time Integrator1/1 -> Sum4/2, Gain3/1
  Sum4/1 -> Out1/1
  Gain4/1 -> Sum4/1

== system exampleMicrogridLibrary/Diesel Generator (Simple Controls)/Discrete/Diesel Engine Governor/TF1 ==
  In1 : Inport
  Discrete-Time Integrator : DiscreteIntegrator  SampleTime=Ts  ICPrevOutput=DiscIntNeverNeededParam  ICPrevScaledInput=DiscIntNeverNeededParam
  Gain : Gain  Gain=1/Ta(2)
  Gain1 : Gain  Gain=Ta(1)
  Sum1 : Sum  Inputs=|+-
  Sum2 : Sum  Inputs=++|
  Out1 : Outport
  wires:
  Gain/1 -> Discrete-Time Integrator/1, Gain1/1
  In1/1 -> Sum1/1
  Discrete-Time Integrator/1 -> Sum2/2, Sum1/2
  Gain1/1 -> Sum2/1
  Sum1/1 -> Gain/1
  Sum2/1 -> Out1/1

== system exampleMicrogridLibrary/Diesel Generator (Simple Controls)/Discrete/Diesel Engine Governor/TF2 ==
  In1 : Inport
  1/T6 : Gain  Gain=1/Ta(3)
  Discrete-Time Integrator : DiscreteIntegrator  SampleTime=Ts  ICPrevOutput=DiscIntNeverNeededParam  ICPrevScaledInput=DiscIntNeverNeededParam
  Sum1 : Sum  Inputs=|+-
  Out1 : Outport
  wires:
  1/T6/1 -> Discrete-Time Integrator/1
  In1/1 -> Sum1/1
  Discrete-Time Integrator/1 -> Out1/1, Sum1/2
  Sum1/1 -> 1/T6/1

== system exampleMicrogridLibrary/Fault /Fault A/Model/Timer ==
  Derivative : Derivative  Commented=on
  Digital Clock : DigitalClock  SampleTime=Ts
  Hit Crossing : HitCross  Commented=on  ShowOutputPort=off
  Look-Up Table : Lookup  InputValues=tv  Table=opv  SaturateOnIntegerOverflow=on
  Out : Outport
  wires:
  Derivative/1 -> Hit Crossing/1
  Look-Up Table/1 -> Derivative/1, Out/1
  Digital Clock/1 -> Look-Up Table/1

== system exampleMicrogridLibrary/Fault /Fault B/Model/Timer ==
  Derivative : Derivative  Commented=on
  Digital Clock : DigitalClock  SampleTime=Ts
  Hit Crossing : HitCross  Commented=on  ShowOutputPort=off
  Look-Up Table : Lookup  InputValues=tv  Table=opv  SaturateOnIntegerOverflow=on
  Out : Outport
  wires:
  Derivative/1 -> Hit Crossing/1
  Look-Up Table/1 -> Derivative/1, Out/1
  Digital Clock/1 -> Look-Up Table/1

== system exampleMicrogridLibrary/Fault /Fault C/Model/Timer ==
  Derivative : Derivative  Commented=on
  Digital Clock : DigitalClock  SampleTime=Ts
  Hit Crossing : HitCross  Commented=on  ShowOutputPort=off
  Look-Up Table : Lookup  InputValues=tv  Table=opv  SaturateOnIntegerOverflow=on
  Out : Outport
  wires:
  Derivative/1 -> Hit Crossing/1
  Look-Up Table/1 -> Derivative/1, Out/1
  Digital Clock/1 -> Look-Up Table/1

== system exampleMicrogridLibrary/Grid-Connected Battery (EMT with Simple Controls)/Inverter Control/Current Control/Current Regulator ==
  note: Id positive --> The converter generates active power ("Inverter mode") = Active Power P positive
  note: Iq positive --> The converter absorbs reactive power ("Inductive mode") = Reactive Power Q negative
  note: Sign Convention: Current going out of the converter = positive current
  note: Current Regulator
      | ================
  VdVq_meas : Inport  PortDimensions=2
  IdIq_meas : Inport  Port=2  PortDimensions=2
  IdIq_ref : Inport  Port=3  PortDimensions=2
  Add1 : Sum  Inputs=++-
  Add2 : Sum
  Add3 : Sum  Inputs=+++
  Demux : Demux  Outputs=2
  Demux1 : Demux  Outputs=2
  Lff : Gain  Gain=Ltot_pu  SaturateOnIntegerOverflow=on  OutDataTypeStr=Inherit: Same as input  ParamDataTypeStr=Inherit: Same as input
  "Lff  " : Gain  Gain=Ltot_pu  SaturateOnIntegerOverflow=on  OutDataTypeStr=Inherit: Same as input  ParamDataTypeStr=Inherit: Same as input
  Mux : Mux  Inputs=2
  PI : simulink/Continuous/PID Controller  Controller=PI  TimeDomain=Discrete-time  SampleTime=Ts_Control  IntegratorMethod=Forward Euler  FilterMethod=Forward Euler  Form=Parallel  UseFilter=on  ControllerParametersSource=internal  P=Kp_Ireg  I=Ki_Ireg  D=0  N=100  InitialConditionSource=internal  InitialConditionForIntegrator=0  InitialConditionForFilter=0  ExternalReset=none  LimitOutput=on  UpperSaturationLimit=1.5  LowerSaturationLimit=-1.5  LinearizeAsGain=off  AntiWindupMode=clamping  Kb=1  TrackingMode=off  Kt=1  PParamMin=[]  PParamMax=[]  IParamMin=[]  IParamMax=[]  DParamMin=[]  DParamMax=[]  NParamMin=[]  NParamMax=[]  KbParamMin=[]  KbParamMax=[]  KtParamMin=[]  KtParamMax=[]  POutMin=[]  POutMax=[]  IOutMin=[]  IOutMax=[]  DOutMin=[]  DOutMax=[]  NOutMin=[]  NOutMax=[]  KbOutMin=[]  KbOutMax=[]  KtOutMin=[]  KtOutMax=[]  IntegratorOutMin=[]  IntegratorOutMax=[]  FilterOutMin=[]  FilterOutMax=[]  SumOutMin=[]  SumOutMax=[]  SumI1OutMin=[]  SumI1OutMax=[]  SumI2OutMin=[]  SumI2OutMax=[]  SumI3OutMin=[]  SumI3OutMax=[]  SumDOutMin=[]  SumDOutMax=[]  SaturationOutMin=[]  SaturationOutMax=[]  IntegratorContinuousStateAttributes=''  IntegratorStateMustResolveToSignalObject=off  IntegratorRTWStateStorageClass=Auto  FilterContinuousStateAttributes=''  FilterStateMustResolveToSignalObject=off  FilterRTWStateStorageClass=Auto  DifferentiatorICPrevScaledInput=0  DifferentiatorOutMin=[]  DifferentiatorOutMax=[]  InitialConditionSetting=State (most efficient)  FilterDiffOutCoefMin=[]  FilterDiffOutCoefMax=[]  SumDenOutMin=[]  SumDenOutMax=[]  SumNumOutMin=[]  SumNumOutMax=[]  ReciprocalOutMin=[]  ReciprocalOutMax=[]  DivideOutMin=[]  DivideOutMax=[]  TunerSelectOption=Transfer Function Based (PID Tuner App)
  Rff : Gain  Gain=Rtot_pu  SaturateOnIntegerOverflow=on  OutDataTypeStr=Inherit: Same as input  ParamDataTypeStr=Inherit: Same as input
  "Rff " : Gain  Gain=Rtot_pu  SaturateOnIntegerOverflow=on  OutDataTypeStr=Inherit: Same as input  ParamDataTypeStr=Inherit: Same as input
  Saturation : Saturate  UpperLimit=1.5  LowerLimit=-1.5
  Scope : Scope  NumInputPorts=2
  Sum : Sum  Inputs=|-+
  VdVq_conv : Outport
  wires:
  Add3/1 -> Mux/2
  Demux/2 -> Add3/1
  Add1/1 -> Mux/1  "Feedforward"
  Lff/1 -> Add3/3
  Rff/1 -> Add3/2
  Demux1/2 -> Rff/1, "Lff  "/1
  "Lff  "/1 -> Add1/3
  Demux1/1 -> Lff/1, "Rff "/1
  "Rff "/1 -> Add1/2
  Demux/1 -> Add1/1
  VdVq_meas/1 -> Demux/1
  Saturation/1 -> VdVq_conv/1
  Add2/1 -> Saturation/1
  IdIq_meas/1 -> Sum/1
  IdIq_ref/1 -> Demux1/1, Sum/2
  Sum/1 -> PI/1, Scope/1
  PI/1 -> Add2/1, Scope/2  "PI"
  Mux/1 -> Add2/2

== system exampleMicrogridLibrary/Grid-Connected Battery (EMT with Simple Controls)/Inverter Control/Current Control/Uabc_ref Generation max (m) = 1 ==
  note: Uref Generation
      | ==============
  note: (Correction for delai of Ts_Control)
  note: (Correction for transformer
      |  D1 connection)
  wt : Inport
  VdVq_conv : Inport  Port=2
  Add1 : Sum  Inputs=++++
  Add2 : Sum
  Complex to Magnitude-Angle : ComplexToMagnitudeAngle
  Constant : Constant  Value=-pi/6
  Constant1 : Constant  Value=Vnom_dc
  Constant2 : Constant  Value="[ 0  -2*pi/3  2*pi/3  ]"
  Constant3 : Constant  Value=Vnom_sec*sqrt(2)/sqrt(3)
  Constant4 : Constant  Value=Ts_Control*Fnom*(2*pi)
  Demux1 : Demux  Outputs=2
  Gain1 : Gain  Gain=1/2
  Product : Product  Inputs=*/  RndMeth=Zero
  Product1 : Product  Inputs=*/  RndMeth=Zero
  Product2 : Product  Inputs=**  RndMeth=Zero
  Real-Imag to Complex : RealImagToComplex
  Trigonometric Function : Trigonometry
  Uabc_ref : Outport
  wires:
  Constant4/1 -> Add1/4
  wt/1 -> Add1/1
  Product2/1 -> Uabc_ref/1
  Trigonometric Function/1 -> Product2/2
  Complex to Magnitude-Angle/1 -> Product2/1
  Add2/1 -> Trigonometric Function/1
  Add1/1 -> Add2/2
  Complex to Magnitude-Angle/2 -> Add2/1
  Product/1 -> Product1/2
  Constant3/1 -> Product/2
  Constant/1 -> Add1/3
  Constant2/1 -> Add1/2
  Demux1/2 -> Real-Imag to Complex/2
  Demux1/1 -> Real-Imag to Complex/1
  Real-Imag to Complex/1 -> Complex to Magnitude-Angle/1
  Gain1/1 -> Product/1
  Product1/1 -> Demux1/1
  VdVq_conv/1 -> Product1/1
  Constant1/1 -> Gain1/1

== system exampleMicrogridLibrary/Grid-Connected Battery (Multi-mode EMT Model)/Inverter Control/Current Control/Current Regulator ==
  note: Current Regulator
      | ================
  note: Sign Convention: Current going out of the converter = positive current
  note: Iq positive --> The converter absorbs reactive power ("Inductive mode") = Reactive Power Q negative
  note: Id positive --> The converter generates active power ("Inverter mode") = Active Power P positive
  VdVq_meas : Inport  PortDimensions=2
  IdIq_meas : Inport  Port=2  PortDimensions=2
  IdIq_ref : Inport  Port=3  PortDimensions=2
  Add1 : Sum  Inputs=++-
  Add2 : Sum
  Add3 : Sum  Inputs=+++
  Demux : Demux  Outputs=2
  Demux1 : Demux  Outputs=2
  Lff : Gain  Gain=Ltot_pu  SaturateOnIntegerOverflow=on  OutDataTypeStr=Inherit: Same as input  ParamDataTypeStr=Inherit: Same as input
  "Lff  " : Gain  Gain=Ltot_pu  SaturateOnIntegerOverflow=on  OutDataTypeStr=Inherit: Same as input  ParamDataTypeStr=Inherit: Same as input
  Mux : Mux  Inputs=2
  PI : simulink/Continuous/PID Controller  Controller=PI  TimeDomain=Discrete-time  SampleTime=Ts_Control  IntegratorMethod=Forward Euler  FilterMethod=Forward Euler  Form=Parallel  UseFilter=on  ControllerParametersSource=internal  P=Kp_Ireg  I=Ki_Ireg  D=0  N=100  InitialConditionSource=internal  InitialConditionForIntegrator=0  InitialConditionForFilter=0  ExternalReset=none  LimitOutput=on  UpperSaturationLimit=1.5  LowerSaturationLimit=-1.5  LinearizeAsGain=off  AntiWindupMode=clamping  Kb=1  TrackingMode=off  Kt=1  PParamMin=[]  PParamMax=[]  IParamMin=[]  IParamMax=[]  DParamMin=[]  DParamMax=[]  NParamMin=[]  NParamMax=[]  KbParamMin=[]  KbParamMax=[]  KtParamMin=[]  KtParamMax=[]  POutMin=[]  POutMax=[]  IOutMin=[]  IOutMax=[]  DOutMin=[]  DOutMax=[]  NOutMin=[]  NOutMax=[]  KbOutMin=[]  KbOutMax=[]  KtOutMin=[]  KtOutMax=[]  IntegratorOutMin=[]  IntegratorOutMax=[]  FilterOutMin=[]  FilterOutMax=[]  SumOutMin=[]  SumOutMax=[]  SumI1OutMin=[]  SumI1OutMax=[]  SumI2OutMin=[]  SumI2OutMax=[]  SumI3OutMin=[]  SumI3OutMax=[]  SumDOutMin=[]  SumDOutMax=[]  SaturationOutMin=[]  SaturationOutMax=[]  IntegratorContinuousStateAttributes=''  IntegratorStateMustResolveToSignalObject=off  IntegratorRTWStateStorageClass=Auto  FilterContinuousStateAttributes=''  FilterStateMustResolveToSignalObject=off  FilterRTWStateStorageClass=Auto  DifferentiatorICPrevScaledInput=0  DifferentiatorOutMin=[]  DifferentiatorOutMax=[]  InitialConditionSetting=State (most efficient)  FilterDiffOutCoefMin=[]  FilterDiffOutCoefMax=[]  SumDenOutMin=[]  SumDenOutMax=[]  SumNumOutMin=[]  SumNumOutMax=[]  ReciprocalOutMin=[]  ReciprocalOutMax=[]  DivideOutMin=[]  DivideOutMax=[]  TunerSelectOption=Transfer Function Based (PID Tuner App)
  Rff : Gain  Gain=Rtot_pu  SaturateOnIntegerOverflow=on  OutDataTypeStr=Inherit: Same as input  ParamDataTypeStr=Inherit: Same as input
  "Rff " : Gain  Gain=Rtot_pu  SaturateOnIntegerOverflow=on  OutDataTypeStr=Inherit: Same as input  ParamDataTypeStr=Inherit: Same as input
  Saturation : Saturate  UpperLimit=1.5  LowerLimit=-1.5
  Scope : Scope  NumInputPorts=2
  Sum : Sum  Inputs=|-+
  VdVq_conv : Outport
  wires:
  Mux/1 -> Add2/2
  PI/1 -> Scope/2, Add2/1  "PI"
  Sum/1 -> Scope/1, PI/1
  IdIq_ref/1 -> Sum/2, Demux1/1
  IdIq_meas/1 -> Sum/1
  Add2/1 -> Saturation/1
  Saturation/1 -> VdVq_conv/1
  VdVq_meas/1 -> Demux/1
  Demux/1 -> Add1/1
  "Rff "/1 -> Add1/2
  Demux1/1 -> "Rff "/1, Lff/1
  "Lff  "/1 -> Add1/3
  Demux1/2 -> "Lff  "/1, Rff/1
  Rff/1 -> Add3/2
  Lff/1 -> Add3/3
  Add1/1 -> Mux/1  "Feedforward"
  Demux/2 -> Add3/1
  Add3/1 -> Mux/2

== system exampleMicrogridLibrary/Grid-Connected Battery (Multi-mode EMT Model)/Inverter Control/Current Control/Uabc_ref Generation max (m) = 1 ==
  note: (Correction for transformer
      |  D1 connection)
  note: (Correction for delai of Ts_Control)
  note: Uref Generation
      | ==============
  wt : Inport
  VdVq_conv : Inport  Port=2
  Add1 : Sum  Inputs=++++
  Add2 : Sum
  Complex to Magnitude-Angle : ComplexToMagnitudeAngle
  Constant : Constant  Value=-pi/6
  Constant1 : Constant  Value=Vnom_dc
  Constant2 : Constant  Value="[ 0  -2*pi/3  2*pi/3  ]"
  Constant3 : Constant  Value=Vnom_sec*sqrt(2)/sqrt(3)
  Constant4 : Constant  Value=Ts_Control*Fnom*(2*pi)
  Demux1 : Demux  Outputs=2
  Gain1 : Gain  Gain=1/2
  Product : Product  Inputs=*/  RndMeth=Zero
  Product1 : Product  Inputs=*/  RndMeth=Zero
  Product2 : Product  Inputs=**  RndMeth=Zero
  Real-Imag to Complex : RealImagToComplex
  Trigonometric Function : Trigonometry
  Uabc_ref : Outport
  wires:
  Constant1/1 -> Gain1/1
  VdVq_conv/1 -> Product1/1
  Product1/1 -> Demux1/1
  Gain1/1 -> Product/1
  Real-Imag to Complex/1 -> Complex to Magnitude-Angle/1
  Demux1/1 -> Real-Imag to Complex/1
  Demux1/2 -> Real-Imag to Complex/2
  Constant2/1 -> Add1/2
  Constant/1 -> Add1/3
  Constant3/1 -> Product/2
  Product/1 -> Product1/2
  Complex to Magnitude-Angle/2 -> Add2/1
  Add1/1 -> Add2/2
  Add2/1 -> Trigonometric Function/1
  Complex to Magnitude-Angle/1 -> Product2/1
  Trigonometric Function/1 -> Product2/2
  Product2/1 -> Uabc_ref/1
  wt/1 -> Add1/1
  Constant4/1 -> Add1/4

== system exampleMicrogridLibrary/Power Equation Wind Turbine (PQ Model)/Wind Turbine Power Equation/Wind Turbine Properties/Properties ==
  In1 : Inport
  Air Density : Gain  Gain=rho
  Blade Swept Area (m^2) : Gain  Gain=A
  Gain : Gain  Gain=1/2
  Power Coefficient : Constant  Value=Cp
  "Product " : Product  SaturateOnIntegerOverflow=on  OutDataTypeStr=Inherit: Same as first input
  wind_speed^3 : Fcn  Expr=u(1)^3
  Out1 : Outport
  wires:
  Blade Swept Area (m^2)/1 -> "Product "/1
  wind_speed^3/1 -> Air Density/1
  Power Coefficient/1 -> "Product "/2
  In1/1 -> wind_speed^3/1
  Air Density/1 -> Gain/1
  "Product "/1 -> Out1/1
  Gain/1 -> Blade Swept Area (m^2)/1

== system exampleMicrogridLibrary/Relay/Breaker (Pure Discrete)/Breaker A/Model ==
  "gate " : Inport
  Uswitch : Inport  Port=2
  C4 : Constant  Value=BR.com
  Data Type Conversion : DataTypeConversion  OutDataTypeStr=double  SaturateOnIntegerOverflow=on  RndMeth=Zero
  Switch3 : Switch  Threshold=0.5  ZeroCross=off  InputSameDT=on
  This signal is not used : Terminator
  Timer : Subsystem  DialogController=POWERSYS.PowerSysDialog  mask(Timer){t=BR.SwitchingTimes, e=BR.switchings}
      mask prompts: t "Time (s):"; e "Amplitude:"
      mask help:
      | Generates a signal changing at specified times.
      |
      | If a signal value is not specified at time zero, the output is kept at 0 until the first specified transition time.
      mask init: same as exampleMicrogridLibrary/Fault /Fault A/Model/Timer
      mask Help: helpview(psbhelp)
      mask Display: plot( tv(2:end-1), opv(2:end-1) )
  gate : Outport
  wires:
  Uswitch/1 -> This signal is not used/1
  C4/1 -> Switch3/2
  Timer/1(Out) -> Switch3/3
  Data Type Conversion/1 -> Switch3/1
  Switch3/1 -> gate/1
  "gate "/1 -> Data Type Conversion/1

== system exampleMicrogridLibrary/Relay/Breaker (Pure Discrete)/Breaker B/Model ==
  "gate " : Inport
  Uswitch : Inport  Port=2
  C4 : Constant  Value=BR.com
  Data Type Conversion : DataTypeConversion  OutDataTypeStr=double  SaturateOnIntegerOverflow=on  RndMeth=Zero
  Switch3 : Switch  Threshold=0.5  ZeroCross=off  InputSameDT=on
  This signal is not used : Terminator
  Timer : Subsystem  DialogController=POWERSYS.PowerSysDialog  mask(Timer){t=BR.SwitchingTimes, e=BR.switchings}
      mask prompts: t "Time (s):"; e "Amplitude:"
      mask help:
      | Generates a signal changing at specified times.
      |
      | If a signal value is not specified at time zero, the output is kept at 0 until the first specified transition time.
      mask init: same as exampleMicrogridLibrary/Fault /Fault A/Model/Timer
      mask Help: helpview(psbhelp)
      mask Display: plot( tv(2:end-1), opv(2:end-1) )
  gate : Outport
  wires:
  Uswitch/1 -> This signal is not used/1
  C4/1 -> Switch3/2
  Timer/1(Out) -> Switch3/3
  Data Type Conversion/1 -> Switch3/1
  Switch3/1 -> gate/1
  "gate "/1 -> Data Type Conversion/1

== system exampleMicrogridLibrary/Relay/Breaker (Pure Discrete)/Breaker C/Model ==
  "gate " : Inport
  Uswitch : Inport  Port=2
  C4 : Constant  Value=BR.com
  Data Type Conversion : DataTypeConversion  OutDataTypeStr=double  SaturateOnIntegerOverflow=on  RndMeth=Zero
  Switch3 : Switch  Threshold=0.5  ZeroCross=off  InputSameDT=on
  This signal is not used : Terminator
  Timer : Subsystem  DialogController=POWERSYS.PowerSysDialog  mask(Timer){t=BR.SwitchingTimes, e=BR.switchings}
      mask prompts: t "Time (s):"; e "Amplitude:"
      mask help:
      | Generates a signal changing at specified times.
      |
      | If a signal value is not specified at time zero, the output is kept at 0 until the first specified transition time.
      mask init: same as exampleMicrogridLibrary/Fault /Fault A/Model/Timer
      mask Help: helpview(psbhelp)
      mask Display: plot( tv(2:end-1), opv(2:end-1) )
  gate : Outport
  wires:
  Uswitch/1 -> This signal is not used/1
  C4/1 -> Switch3/2
  Timer/1(Out) -> Switch3/3
  Data Type Conversion/1 -> Switch3/1
  Switch3/1 -> gate/1
  "gate "/1 -> Data Type Conversion/1

== system exampleMicrogridLibrary/SPS-Simulink Interface/EMT/Frequency Generator/Continuous ==
  Clock : Clock
  Constant4 : Constant  Value=2*pi
  Freq1 : Constant  Value=Freq
  Freq2 : Constant  Value=2*pi
  Math Function : Math  Operator=mod  SaturateOnIntegerOverflow=on
  Product3 : Product  Inputs=***  SaturateOnIntegerOverflow=on  InputSameDT=on  OutDataTypeStr=Inherit: Same as first input
  2pi*f : Outport
  wires:
  Clock/1 -> Product3/2
  Freq2/1 -> Product3/3
  Freq1/1 -> Product3/1
  Constant4/1 -> Math Function/2
  Product3/1 -> Math Function/1
  Math Function/1 -> 2pi*f/1

== system exampleMicrogridLibrary/SPS-Simulink Interface/EMT/Frequency Generator/Discrete ==
  Constant4 : Constant  Value=2*pi
  Freq1 : Constant  Value=Freq
  Freq2 : Constant  Value=2*pi
  Math Function : Math  Operator=mod  SaturateOnIntegerOverflow=on
  Product3 : Product  Inputs=***  SaturateOnIntegerOverflow=on  InputSameDT=on  OutDataTypeStr=Inherit: Same as first input
  t : DigitalClock  SampleTime=Ts
  2pi*f : Outport
  wires:
  Math Function/1 -> 2pi*f/1
  Product3/1 -> Math Function/1
  Constant4/1 -> Math Function/2
  Freq1/1 -> Product3/1
  Freq2/1 -> Product3/3
  t/1 -> Product3/2

== system exampleMicrogridLibrary/Relay/Breaker (Pure Discrete)/Breaker A/Model/Timer ==
  Derivative : Derivative  Commented=on
  Digital Clock : DigitalClock  SampleTime=Ts
  Hit Crossing : HitCross  Commented=on  ShowOutputPort=off
  Look-Up Table : Lookup  InputValues=tv  Table=opv  SaturateOnIntegerOverflow=on
  Out : Outport
  wires:
  Derivative/1 -> Hit Crossing/1
  Look-Up Table/1 -> Derivative/1, Out/1
  Digital Clock/1 -> Look-Up Table/1

== system exampleMicrogridLibrary/Relay/Breaker (Pure Discrete)/Breaker B/Model/Timer ==
  Derivative : Derivative  Commented=on
  Digital Clock : DigitalClock  SampleTime=Ts
  Hit Crossing : HitCross  Commented=on  ShowOutputPort=off
  Look-Up Table : Lookup  InputValues=tv  Table=opv  SaturateOnIntegerOverflow=on
  Out : Outport
  wires:
  Derivative/1 -> Hit Crossing/1
  Look-Up Table/1 -> Derivative/1, Out/1
  Digital Clock/1 -> Look-Up Table/1

== system exampleMicrogridLibrary/Relay/Breaker (Pure Discrete)/Breaker C/Model/Timer ==
  Derivative : Derivative  Commented=on
  Digital Clock : DigitalClock  SampleTime=Ts
  Hit Crossing : HitCross  Commented=on  ShowOutputPort=off
  Look-Up Table : Lookup  InputValues=tv  Table=opv  SaturateOnIntegerOverflow=on
  Out : Outport
  wires:
  Derivative/1 -> Hit Crossing/1
  Look-Up Table/1 -> Derivative/1, Out/1
  Digital Clock/1 -> Look-Up Table/1

== matlab function exampleMicrogridLibrary/Solar Array (EMT Model)/Inverter Control/MPPT Controller using Perturbe & Observe technique  ==
  settings: updateMethod=DISCRETE  sampleTime=Ts_Control
  data: Param input; Enabled input; V input =V; I input; D output
function D  = PandO(Param, Enabled, V, I)

% MPPT controller based on the Perturb & Observe algorithm.

% D output = Reference for DC link voltage (Vdc_ref) 
%
% Enabled input = 1 to enable the MPPT controller
% V input = PV array terminal voltage (V)
% I input = PV array current (A)
%
% Param input:
Dinit = Param(1);  %Initial value for Vdc_ref
Dmax = Param(2);   %Maximum value for Vdc_ref
Dmin = Param(3);   %Minimum value for Vdc_ref
deltaD = Param(4); %Increment value used to increase/decrease Vdc_ref
%  

persistent Vold Pold Dold;

dataType = 'double';

if isempty(Vold)
    Vold=0;
    Pold=0;
    Dold=Dinit;
end
P= V*I;
dV= V - Vold;
dP= P - Pold;

if dP ~= 0 & Enabled ~=0
    if dP < 0
        if dV < 0
            D = Dold + deltaD;
        else
            D = Dold - deltaD;
        end
    else
        if dV < 0
            D = Dold - deltaD;
        else
            D = Dold + deltaD;
        end    
    end
else D=Dold;
end

if D >= Dmax | D<= Dmin
    D=Dold;
end

Dold=D;
Vold=V;
Pold=P;
